simulink model "Beo_I_nichtlinear"  (R2019a)
settings: Solver=VariableStepAuto  StartTime=0.0  StopTime=10.0  RelTol=1e-3
values from neighbouring files (symbols this model uses):
  A = [0 1 0 0;m*g*l(M+m)/d 0 0 m*l*b/d;0 0 0 1;-g*m^2*l^2/d 0 0 -b*(I+m*l^2)/d]    [inv_pend.m]
  B = [0;-m*l/d;0;(I+m*l^2)/d]    [inv_pend.m]
  b = 0.1    [inv_pend.m]
  C = [0 0 1 0;1 0 0 0]    [inv_pend.m]
  d = I*(M+m)+M*m*l^2    (= 0.0285)    [inv_pend.m]
  g = 9.8    [inv_pend.m]
  I = 0.006    [inv_pend.m]
  K1 = KI(:,1:end-size(Cn,1))    [inv_pend.m]
  K2 = KI(:,end-size(Cn,1)+1:end)    [inv_pend.m]
  L = place(A',C',[-30 -31 -32 -33])'    [inv_pend.m]
  l = 0.3    [inv_pend.m]
  m = 0.5    [inv_pend.m]
  M = 0.5    [inv_pend.m]
settings Model: Creator=Naveen  LastModifiedBy=Naveen

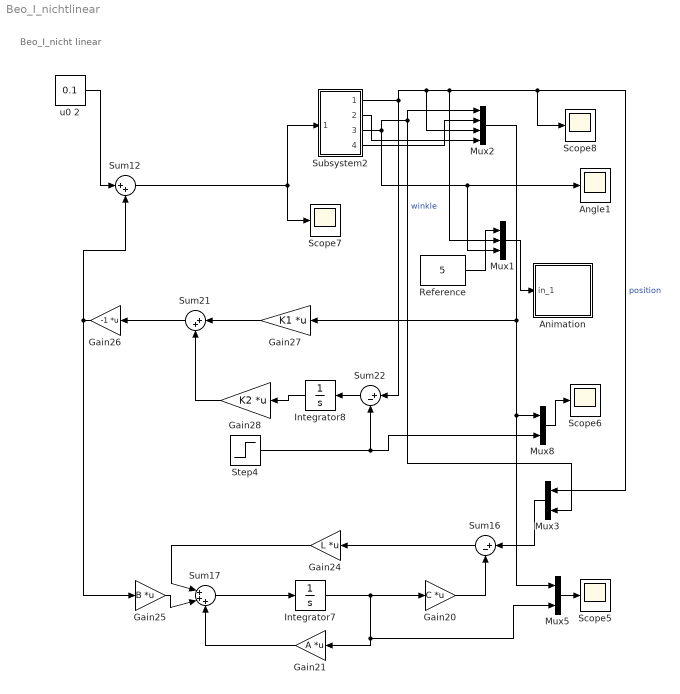
== system Beo_I_nichtlinear ==
  note: Beo_I_nicht linear
  Angle1 : Scope
  Animation : Subsystem  mask(Pendulum plot){RefBlock=Reference}
      mask prompts: RefBlock "DC reference signal block name:"
      mask help: Pendulum plot
      mask Help: Pendulum animation function using Handle graphics.
      mask Display: plot([-10 10],[0 0],[-2 -2 2 2],[0 1 1 0],[0 3],[1 5])
  Gain20 : Gain  Gain=C  Multiplication=Matrix(K*u)
  Gain21 : Gain  Gain=A  Multiplication=Matrix(K*u)
  Gain24 : Gain  Gain=L  Multiplication=Matrix(K*u)
  Gain25 : Gain  Gain=B  Multiplication=Matrix(K*u)
  Gain26 : Gain  Gain=-1  Multiplication=Matrix(K*u)
  Gain27 : Gain  Gain=K1  Multiplication=Matrix(K*u)
  Gain28 : Gain  Gain=K2  Multiplication=Matrix(K*u)
  Integrator7 : Integrator
  Integrator8 : Integrator
  Mux1 : Mux  Inputs=3
  Mux2 : Mux
  Mux3 : Mux  Inputs=2
  Mux5 : Mux  Inputs=2
  Mux8 : Mux  Inputs=2
  Reference : Constant  Value=5
  Scope{5..8} (4 alike) : Scope
  Step4 : Step  Time=0  After=5  SampleTime=0
  Subsystem2 : Subsystem
  Sum12 : Sum  Inputs=|++
  Sum16 : Sum  Inputs=|+-
  Sum17 : Sum  Inputs=|+++
  Sum21 : Sum  Inputs=|++
  Sum22 : Sum  Inputs=|+-
  u0 2 : Constant  Value=0.1
  wires:
  Gain27/1 -> Sum21/1
  Gain20/1 -> Sum16/2
  Integrator8/1 -> Gain28/1
  Step4/1 -> Mux8/2, Sum22/2
  Sum12/1 -> Subsystem2/1(Force), Scope7/1
  Sum22/1 -> Integrator8/1
  u0 2/1 -> Sum12/1
  Gain24/1 -> Sum17/1
  Mux3/1 -> Sum16/1
  Mux2/1 -> Gain27/1, Mux8/1, Mux5/1
  Sum21/1 -> Gain26/1
  Gain21/1 -> Sum17/3
  Integrator7/1 -> Mux5/2, Gain21/1, Gain20/1
  Mux8/1 -> Scope6/1
  Gain28/1 -> Sum21/2
  Gain26/1 -> Sum12/2, Gain25/1
  Subsystem2/4(thetadot) -> Mux2/2
  Sum17/1 -> Integrator7/1
  Sum16/1 -> Gain24/1
  Subsystem2/2(xdot) -> Mux2/4
  Gain25/1 -> Sum17/2
  Mux5/1 -> Scope5/1
  Subsystem2/1(Position) -> Mux2/3, Mux1/2, Scope8/1, Mux3/1, Sum22/1  "position"
  Subsystem2/3(Angle) -> Mux2/1, Mux3/2, Mux1/3, Angle1/1  "winkle"
  Reference/1 -> Mux1/1
  Mux1/1 -> Animation/1(in_1)

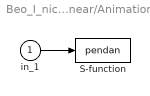
== system Beo_I_nichtlinear/Animation ==
  in_1 : Inport
  S-function : S-Function  FunctionName=pendan  Parameters=RefBlock  SFunctionDeploymentMode=off  EnableBusSupport=off
      settings: DeleteFcn=pendan([],[],[],'DeleteBlock');
  wires:
  in_1/1 -> S-function/1

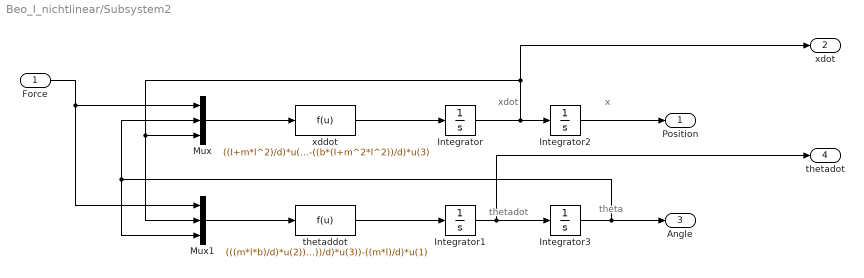
== system Beo_I_nichtlinear/Subsystem2 ==
  note: x
  note: thetadot
  note: theta
  note: xdot
  Force : Inport
  Integrator : Integrator  ContinuousStateAttributes='xdot'
  Integrator1 : Integrator  ContinuousStateAttributes='thetadot'
  Integrator2 : Integrator  ContinuousStateAttributes='x'
  Integrator3 : Integrator  ContinuousStateAttributes='theta'
  Mux : Mux  Inputs=3
  Mux1 : Mux  Inputs=3
  thetaddot : Fcn  Expr=(((m*l*b)/d)*u(2))+(((m*g*l*(M+m))/d)*u(3))-((m*l)/d)*u(1)
  xddot : Fcn  Expr=((I+m*l^2)/d)*u(1)-((g*m^2*l^2)/d)*u(2)-((b*(I+m^2*l^2))/d)*u(3)
  Position : Outport
  xdot : Outport  Port=2
  Angle : Outport  Port=3
  thetadot : Outport  Port=4
  wires:
  Integrator2/1 -> Position/1
  Integrator3/1 -> Mux/2, Mux1/3, Angle/1
  Force/1 -> Mux1/1, Mux/1
  Integrator1/1 -> thetadot/1, Integrator3/1
  xddot/1 -> Integrator/1
  Integrator/1 -> xdot/1, Mux1/2, Mux/3, Integrator2/1
  Mux1/1 -> thetaddot/1
  Mux/1 -> xddot/1
  thetaddot/1 -> Integrator1/1
